simulink model "IC74181Model"  (R2022b)
settings: Solver=VariableStepAuto  StartTime=0.0  StopTime=10.0  RelTol=1e-3
settings Model: Creator=OmerFarukCanbaz  LastModifiedBy=OmerFarukCanbaz

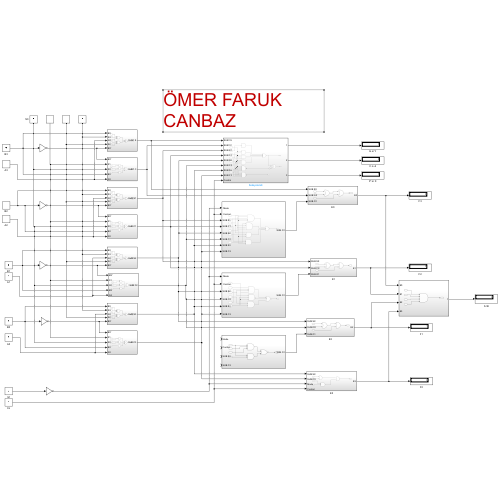
[thumbnail: Simulink's stored preview of the top-level diagram]
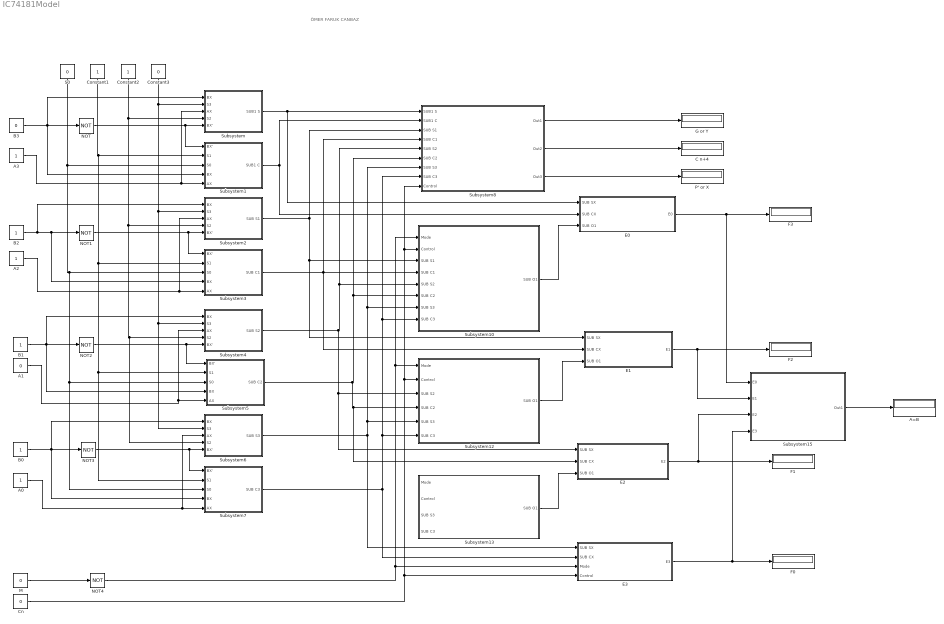
== system IC74181Model ==
  note: ÖMER FARUK CANBAZ
  A0 : Constant
  A1 : Constant  Value=0
  A2 : Constant
  A3 : Constant
  A=B : Display
  B0 : Constant
  B1 : Constant
  B2 : Constant
  B3 : Constant  Value=0
  C n+4 : Display
  Cn : Constant  Value=0
  Constant1 : Constant
  Constant2 : Constant
  Constant3 : Constant  Value=0
  E0 : Subsystem
  E1 : Subsystem
  E2 : Subsystem
  E3 : Subsystem
  F{0..3} (4 alike) : Display
  G or Y : Display
  M : Constant  Value=0
  NOT{,1..4} (5 alike) : Logic  Operator=NOT  IconShape=distinctive  AllPortsSameDT=off  OutDataTypeStr=boolean
  P' or X : Display
  S0 : Constant  Value=0
  Subsystem : Subsystem
  Subsystem1 : Subsystem
  Subsystem10 : Subsystem
  Subsystem12 : Subsystem
  Subsystem13 : Subsystem
  Subsystem15 : Subsystem
  Subsystem2 : Subsystem
  Subsystem3 : Subsystem
  Subsystem4 : Subsystem
  Subsystem5 : Subsystem
  Subsystem6 : Subsystem
  Subsystem7 : Subsystem
  Subsystem8 : Subsystem
  wires:
  B3/1 -> Subsystem/1(BX), NOT/1, Subsystem1/4(BX)
  NOT/1 -> Subsystem1/1(BX'), Subsystem/5(BX')
  A3/1 -> Subsystem/3(AX), Subsystem1/5(AX)
  NOT1/1 -> Subsystem3/1(BX'), Subsystem2/5(BX')
  NOT2/1 -> Subsystem5/1(BX'), Subsystem4/5(BX')
  NOT3/1 -> Subsystem7/1(BX'), Subsystem6/5(BX')
  B2/1 -> Subsystem3/4(BX), NOT1/1, Subsystem2/1(BX)
  A2/1 -> Subsystem2/3(AX), Subsystem3/5(AX)
  B1/1 -> NOT2/1, Subsystem5/4(BX), Subsystem4/1(BX)
  A1/1 -> Subsystem4/3(AX), Subsystem5/5(AX)
  B0/1 -> Subsystem7/4(BX), Subsystem6/1(BX), NOT3/1
  A0/1 -> Subsystem6/3(AX), Subsystem7/5(AX)
  Constant3/1 -> Subsystem6/2(S3), Subsystem4/2(S3), Subsystem2/2(S3), Subsystem/2(S3)
  Constant2/1 -> Subsystem6/4(S2), Subsystem4/4(S2), Subsystem2/4(S2), Subsystem/4(S2)
  Constant1/1 -> Subsystem7/2(S1), Subsystem5/2(S1), Subsystem3/2(S1), Subsystem1/2(S1)
  S0/1 -> Subsystem7/3(S0), Subsystem5/3(S0), Subsystem3/3(S0), Subsystem1/3(S0)
  Subsystem8/1(Out1) -> G or Y/1
  Subsystem8/2(Out2) -> C n+4/1
  Subsystem8/3(Out3) -> P' or X/1
  Subsystem/1(SUB1 S) -> E0/1(SUB SX), Subsystem8/1(SUB1 S)
  Subsystem1/1(SUB1 C) -> Subsystem8/2(SUB1 C), E0/2(SUB CX)
  Subsystem2/1(SUB S1) -> E1/1(SUB SX), Subsystem10/3(SUB S1), Subsystem8/3(SUB S1)
  Subsystem3/1(SUB C1) -> E1/2(SUB CX), Subsystem8/4(SUB C1), Subsystem10/4(SUB C1)
  Subsystem4/1(SUB S2) -> E2/1(SUB SX), Subsystem12/3(SUB S2), Subsystem8/5(SUB S2), Subsystem10/5(SUB S2)
  Subsystem5/1(SUB C2) -> E2/2(SUB CX), Subsystem12/4(SUB C2), Subsystem8/6(SUB C2), Subsystem10/6(SUB C2)
  Subsystem6/1(SUB S3) -> E3/1(SUB SX), Subsystem8/7(SUB S3), Subsystem10/7(SUB S3), Subsystem12/5(SUB S3)
  Subsystem7/1(SUB C3) -> Subsystem12/6(SUB C3), Subsystem8/8(SUB C3), Subsystem10/8(SUB C3), E3/2(SUB CX)
  Cn/1 -> E3/4(Control), Subsystem8/9(Control), Subsystem10/2(" Control"), Subsystem12/2(" Control")
  Subsystem10/1(SUB O1) -> E0/3(SUB O1)
  M/1 -> NOT4/1
  E0/1(E0) -> F3/1, Subsystem15/1(E0)
  NOT4/1 -> E3/3(Mode), Subsystem12/1(" Mode"), Subsystem10/1(" Mode")
  Subsystem12/1(SUB O1) -> E1/3(SUB O1)
  E1/1(E1) -> Subsystem15/2(E1), F2/1
  Subsystem13/1(SUB O1) -> E2/3(SUB O1)
  E2/1(E2) -> F1/1, Subsystem15/3(E2)
  E3/1(E3) -> Subsystem15/4(E3), F0/1
  Subsystem15/1(Out1) -> A=B/1

== system IC74181Model/E0 ==
  SUB SX : Inport
  SUB CX : Inport  Port=2
  SUB O1 : Inport  Port=3
  XOR : Logic  Operator=XOR  IconShape=distinctive  AllPortsSameDT=off  OutDataTypeStr=boolean
  XOR1 : Logic  Operator=XOR  IconShape=distinctive  AllPortsSameDT=off  OutDataTypeStr=boolean
  E0 : Outport
  wires:
  SUB CX/1 -> XOR/2
  SUB SX/1 -> XOR/1
  XOR/1 -> XOR1/1
  SUB O1/1 -> XOR1/2
  XOR1/1 -> E0/1

== system IC74181Model/E1 ==
  SUB SX : Inport
  SUB CX : Inport  Port=2
  SUB O1 : Inport  Port=3
  XOR : Logic  Operator=XOR  IconShape=distinctive  AllPortsSameDT=off  OutDataTypeStr=boolean
  XOR1 : Logic  Operator=XOR  IconShape=distinctive  AllPortsSameDT=off  OutDataTypeStr=boolean
  E1 : Outport
  wires:
  SUB CX/1 -> XOR/2
  SUB SX/1 -> XOR/1
  XOR/1 -> XOR1/1
  SUB O1/1 -> XOR1/2
  XOR1/1 -> E1/1

== system IC74181Model/E2 ==
  SUB SX : Inport
  SUB CX : Inport  Port=2
  SUB O1 : Inport  Port=3
  XOR : Logic  Operator=XOR  IconShape=distinctive  AllPortsSameDT=off  OutDataTypeStr=boolean
  XOR1 : Logic  Operator=XOR  IconShape=distinctive  AllPortsSameDT=off  OutDataTypeStr=boolean
  E2 : Outport
  wires:
  SUB CX/1 -> XOR/2
  SUB SX/1 -> XOR/1
  XOR/1 -> XOR1/1
  SUB O1/1 -> XOR1/2
  XOR1/1 -> E2/1

== system IC74181Model/E3 ==
  SUB SX : Inport
  SUB CX : Inport  Port=2
  Mode : Inport  Port=3
  Control : Inport  Port=4
  NAND : Logic  Operator=NAND  IconShape=distinctive  AllPortsSameDT=off  OutDataTypeStr=boolean
  XOR : Logic  Operator=XOR  IconShape=distinctive  AllPortsSameDT=off  OutDataTypeStr=boolean
  XOR1 : Logic  Operator=XOR  IconShape=distinctive  AllPortsSameDT=off  OutDataTypeStr=boolean
  E3 : Outport
  wires:
  SUB CX/1 -> XOR/2
  SUB SX/1 -> XOR/1
  XOR/1 -> XOR1/1
  Mode/1 -> NAND/1
  XOR1/1 -> E3/1
  Control/1 -> NAND/2
  NAND/1 -> XOR1/2

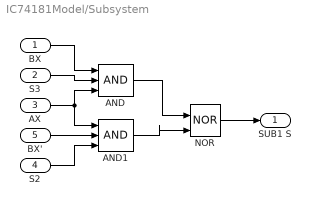
== system IC74181Model/Subsystem ==
  BX : Inport
  S3 : Inport  Port=2
  AX : Inport  Port=3
  S2 : Inport  Port=4
  BX' : Inport  Port=5
  AND : Logic  Inputs=3  IconShape=distinctive  AllPortsSameDT=off  OutDataTypeStr=boolean
  AND1 : Logic  Inputs=3  IconShape=distinctive  AllPortsSameDT=off  OutDataTypeStr=boolean
  NOR : Logic  Operator=NOR  IconShape=distinctive  AllPortsSameDT=off  OutDataTypeStr=boolean
  SUB1 S : Outport
  wires:
  NOR/1 -> SUB1 S/1
  AND1/1 -> NOR/2
  AND/1 -> NOR/1
  AX/1 -> AND1/1, AND/3
  S3/1 -> AND/2
  BX/1 -> AND/1
  S2/1 -> AND1/3
  BX'/1 -> AND1/2

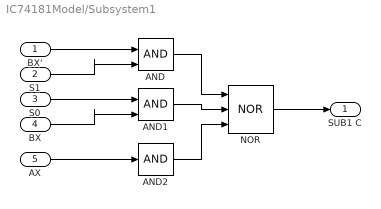
== system IC74181Model/Subsystem1 ==
  BX' : Inport
  S1 : Inport  Port=2
  S0 : Inport  Port=3
  BX : Inport  Port=4
  AX : Inport  Port=5
  AND : Logic  IconShape=distinctive  AllPortsSameDT=off  OutDataTypeStr=boolean
  AND1 : Logic  IconShape=distinctive  AllPortsSameDT=off  OutDataTypeStr=boolean
  AND2 : Logic  Inputs=1  IconShape=distinctive  AllPortsSameDT=off  OutDataTypeStr=boolean
  NOR : Logic  Operator=NOR  Inputs=3  IconShape=distinctive  AllPortsSameDT=off  OutDataTypeStr=boolean
  SUB1 C : Outport
  wires:
  NOR/1 -> SUB1 C/1
  AND/1 -> NOR/1
  AND1/1 -> NOR/2
  AND2/1 -> NOR/3
  AX/1 -> AND2/1
  S0/1 -> AND1/1
  BX/1 -> AND1/2
  S1/1 -> AND/2
  BX'/1 -> AND/1

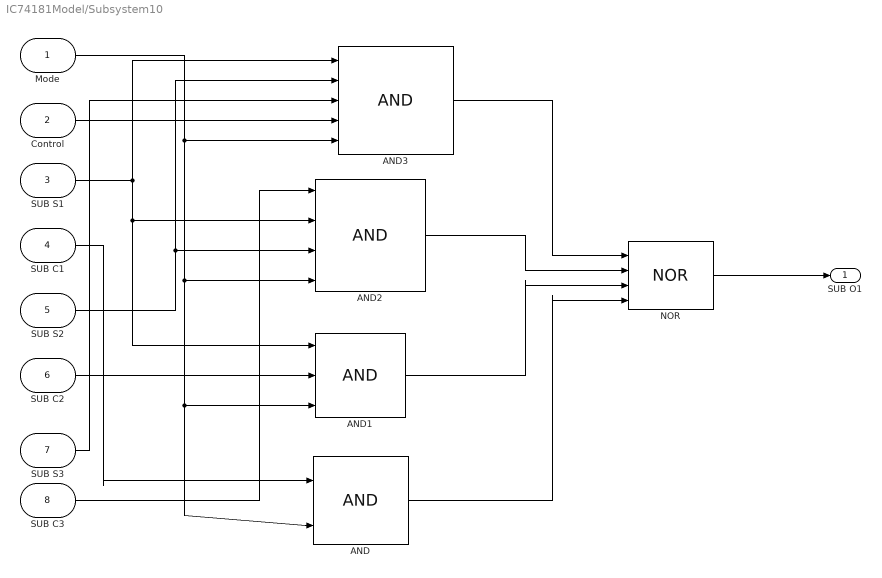
== system IC74181Model/Subsystem10 ==
  " Mode" : Inport
  " Control" : Inport  Port=2
  SUB S1 : Inport  Port=3
  SUB C1 : Inport  Port=4
  SUB S2 : Inport  Port=5
  SUB C2 : Inport  Port=6
  SUB S3 : Inport  Port=7
  SUB C3 : Inport  Port=8
  AND : Logic  IconShape=distinctive  AllPortsSameDT=off  OutDataTypeStr=boolean
  AND1 : Logic  Inputs=3  IconShape=distinctive  AllPortsSameDT=off  OutDataTypeStr=boolean
  AND2 : Logic  Inputs=4  IconShape=distinctive  AllPortsSameDT=off  OutDataTypeStr=boolean
  AND3 : Logic  Inputs=5  IconShape=distinctive  AllPortsSameDT=off  OutDataTypeStr=boolean
  NOR : Logic  Operator=NOR  Inputs=4  IconShape=distinctive  AllPortsSameDT=off  OutDataTypeStr=boolean
  SUB O1 : Outport
  wires:
  AND3/1 -> NOR/1
  AND2/1 -> NOR/2
  AND1/1 -> NOR/3
  AND/1 -> NOR/4
  SUB C1/1 -> AND/1
  " Mode"/1 -> AND2/4, AND/2, AND1/3, AND3/5
  " Control"/1 -> AND3/4
  SUB S3/1 -> AND3/3
  SUB S2/1 -> AND3/2, AND2/3
  SUB C2/1 -> AND1/2
  SUB S1/1 -> AND1/1, AND2/2, AND3/1
  SUB C3/1 -> AND2/1
  NOR/1 -> SUB O1/1

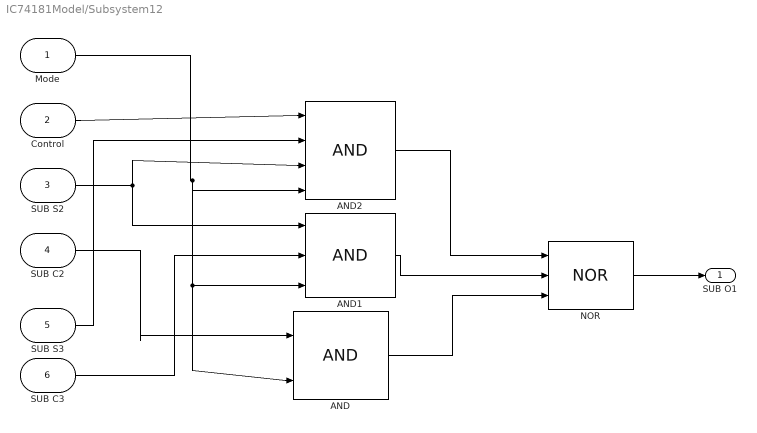
== system IC74181Model/Subsystem12 ==
  " Mode" : Inport
  " Control" : Inport  Port=2
  SUB S2 : Inport  Port=3
  SUB C2 : Inport  Port=4
  SUB S3 : Inport  Port=5
  SUB C3 : Inport  Port=6
  AND : Logic  IconShape=distinctive  AllPortsSameDT=off  OutDataTypeStr=boolean
  AND1 : Logic  Inputs=3  IconShape=distinctive  AllPortsSameDT=off  OutDataTypeStr=boolean
  AND2 : Logic  Inputs=4  IconShape=distinctive  AllPortsSameDT=off  OutDataTypeStr=boolean
  NOR : Logic  Operator=NOR  Inputs=3  IconShape=distinctive  AllPortsSameDT=off  OutDataTypeStr=boolean
  SUB O1 : Outport
  wires:
  NOR/1 -> SUB O1/1
  AND/1 -> NOR/3
  AND1/1 -> NOR/2
  AND2/1 -> NOR/1
  " Mode"/1 -> AND/2, AND1/3, AND2/4
  " Control"/1 -> AND2/1
  SUB S2/1 -> AND1/1, AND2/3
  SUB C2/1 -> AND/1
  SUB C3/1 -> AND1/2
  SUB S3/1 -> AND2/2

== system IC74181Model/Subsystem13 ==
  Mode : Inport
  Control : Inport  Port=2
  SUB S3 : Inport  Port=3
  SUB C3 : Inport  Port=4
  AND : Logic  Inputs=3  IconShape=distinctive  AllPortsSameDT=off  OutDataTypeStr=boolean
  AND1 : Logic  IconShape=distinctive  AllPortsSameDT=off  OutDataTypeStr=boolean
  NOR : Logic  Operator=NOR  IconShape=distinctive  AllPortsSameDT=off  OutDataTypeStr=boolean
  SUB O1 : Outport
  wires:
  Mode/1 -> AND1/1, AND/1
  Control/1 -> AND/2
  SUB S3/1 -> AND/3
  SUB C3/1 -> AND1/2
  NOR/1 -> SUB O1/1
  AND1/1 -> NOR/2
  AND/1 -> NOR/1

== system IC74181Model/Subsystem15 ==
  E0 : Inport
  E1 : Inport  Port=2
  E2 : Inport  Port=3
  E3 : Inport  Port=4
  AND : Logic  Inputs=4  IconShape=distinctive  AllPortsSameDT=off  OutDataTypeStr=boolean
  Out1 : Outport
  wires:
  E3/1 -> AND/4
  E2/1 -> AND/3
  E1/1 -> AND/2
  E0/1 -> AND/1
  AND/1 -> Out1/1

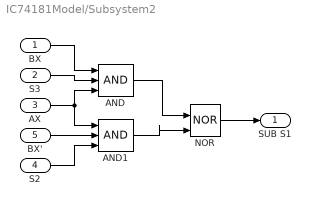
== system IC74181Model/Subsystem2 ==
  BX : Inport
  S3 : Inport  Port=2
  AX : Inport  Port=3
  S2 : Inport  Port=4
  BX' : Inport  Port=5
  AND : Logic  Inputs=3  IconShape=distinctive  AllPortsSameDT=off  OutDataTypeStr=boolean
  AND1 : Logic  Inputs=3  IconShape=distinctive  AllPortsSameDT=off  OutDataTypeStr=boolean
  NOR : Logic  Operator=NOR  IconShape=distinctive  AllPortsSameDT=off  OutDataTypeStr=boolean
  SUB S1 : Outport
  wires:
  NOR/1 -> SUB S1/1
  AND1/1 -> NOR/2
  AND/1 -> NOR/1
  AX/1 -> AND1/1, AND/3
  S3/1 -> AND/2
  BX/1 -> AND/1
  S2/1 -> AND1/3
  BX'/1 -> AND1/2

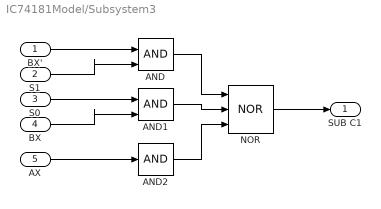
== system IC74181Model/Subsystem3 ==
  BX' : Inport
  S1 : Inport  Port=2
  S0 : Inport  Port=3
  BX : Inport  Port=4
  AX : Inport  Port=5
  AND : Logic  IconShape=distinctive  AllPortsSameDT=off  OutDataTypeStr=boolean
  AND1 : Logic  IconShape=distinctive  AllPortsSameDT=off  OutDataTypeStr=boolean
  AND2 : Logic  Inputs=1  IconShape=distinctive  AllPortsSameDT=off  OutDataTypeStr=boolean
  NOR : Logic  Operator=NOR  Inputs=3  IconShape=distinctive  AllPortsSameDT=off  OutDataTypeStr=boolean
  SUB C1 : Outport
  wires:
  NOR/1 -> SUB C1/1
  AND/1 -> NOR/1
  AND1/1 -> NOR/2
  AND2/1 -> NOR/3
  AX/1 -> AND2/1
  S0/1 -> AND1/1
  BX/1 -> AND1/2
  S1/1 -> AND/2
  BX'/1 -> AND/1

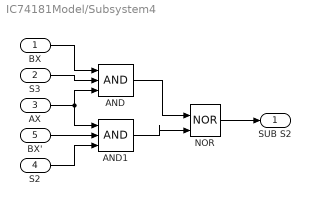
== system IC74181Model/Subsystem4 ==
  BX : Inport
  S3 : Inport  Port=2
  AX : Inport  Port=3
  S2 : Inport  Port=4
  BX' : Inport  Port=5
  AND : Logic  Inputs=3  IconShape=distinctive  AllPortsSameDT=off  OutDataTypeStr=boolean
  AND1 : Logic  Inputs=3  IconShape=distinctive  AllPortsSameDT=off  OutDataTypeStr=boolean
  NOR : Logic  Operator=NOR  IconShape=distinctive  AllPortsSameDT=off  OutDataTypeStr=boolean
  SUB S2 : Outport
  wires:
  NOR/1 -> SUB S2/1
  AND1/1 -> NOR/2
  AND/1 -> NOR/1
  AX/1 -> AND1/1, AND/3
  S3/1 -> AND/2
  BX/1 -> AND/1
  S2/1 -> AND1/3
  BX'/1 -> AND1/2

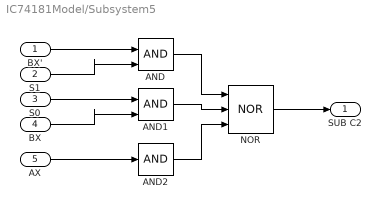
== system IC74181Model/Subsystem5 ==
  BX' : Inport
  S1 : Inport  Port=2
  S0 : Inport  Port=3
  BX : Inport  Port=4
  AX : Inport  Port=5
  AND : Logic  IconShape=distinctive  AllPortsSameDT=off  OutDataTypeStr=boolean
  AND1 : Logic  IconShape=distinctive  AllPortsSameDT=off  OutDataTypeStr=boolean
  AND2 : Logic  Inputs=1  IconShape=distinctive  AllPortsSameDT=off  OutDataTypeStr=boolean
  NOR : Logic  Operator=NOR  Inputs=3  IconShape=distinctive  AllPortsSameDT=off  OutDataTypeStr=boolean
  SUB C2 : Outport
  wires:
  NOR/1 -> SUB C2/1
  AND/1 -> NOR/1
  AND1/1 -> NOR/2
  AND2/1 -> NOR/3
  AX/1 -> AND2/1
  S0/1 -> AND1/1
  BX/1 -> AND1/2
  S1/1 -> AND/2
  BX'/1 -> AND/1

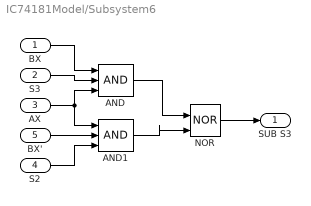
== system IC74181Model/Subsystem6 ==
  BX : Inport
  S3 : Inport  Port=2
  AX : Inport  Port=3
  S2 : Inport  Port=4
  BX' : Inport  Port=5
  AND : Logic  Inputs=3  IconShape=distinctive  AllPortsSameDT=off  OutDataTypeStr=boolean
  AND1 : Logic  Inputs=3  IconShape=distinctive  AllPortsSameDT=off  OutDataTypeStr=boolean
  NOR : Logic  Operator=NOR  IconShape=distinctive  AllPortsSameDT=off  OutDataTypeStr=boolean
  SUB S3 : Outport
  wires:
  NOR/1 -> SUB S3/1
  AND1/1 -> NOR/2
  AND/1 -> NOR/1
  AX/1 -> AND1/1, AND/3
  S3/1 -> AND/2
  BX/1 -> AND/1
  S2/1 -> AND1/3
  BX'/1 -> AND1/2

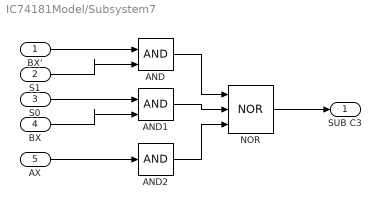
== system IC74181Model/Subsystem7 ==
  BX' : Inport
  S1 : Inport  Port=2
  S0 : Inport  Port=3
  BX : Inport  Port=4
  AX : Inport  Port=5
  AND : Logic  IconShape=distinctive  AllPortsSameDT=off  OutDataTypeStr=boolean
  AND1 : Logic  IconShape=distinctive  AllPortsSameDT=off  OutDataTypeStr=boolean
  AND2 : Logic  Inputs=1  IconShape=distinctive  AllPortsSameDT=off  OutDataTypeStr=boolean
  NOR : Logic  Operator=NOR  Inputs=3  IconShape=distinctive  AllPortsSameDT=off  OutDataTypeStr=boolean
  SUB C3 : Outport
  wires:
  NOR/1 -> SUB C3/1
  AND/1 -> NOR/1
  AND1/1 -> NOR/2
  AND2/1 -> NOR/3
  AX/1 -> AND2/1
  S0/1 -> AND1/1
  BX/1 -> AND1/2
  S1/1 -> AND/2
  BX'/1 -> AND/1

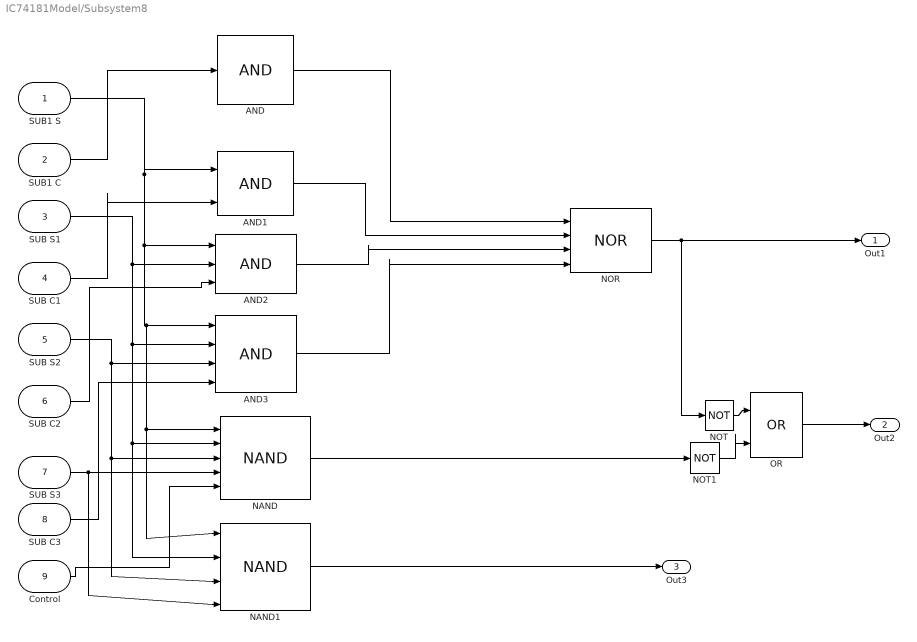
== system IC74181Model/Subsystem8 ==
  SUB1 S : Inport
  SUB1 C : Inport  Port=2
  SUB S1 : Inport  Port=3
  SUB C1 : Inport  Port=4
  SUB S2 : Inport  Port=5
  SUB C2 : Inport  Port=6
  SUB S3 : Inport  Port=7
  SUB C3 : Inport  Port=8
  Control : Inport  Port=9
  AND : Logic  Inputs=1  IconShape=distinctive  AllPortsSameDT=off  OutDataTypeStr=boolean
  AND1 : Logic  IconShape=distinctive  AllPortsSameDT=off  OutDataTypeStr=boolean
  AND2 : Logic  Inputs=3  IconShape=distinctive  AllPortsSameDT=off  OutDataTypeStr=boolean
  AND3 : Logic  Inputs=4  IconShape=distinctive  AllPortsSameDT=off  OutDataTypeStr=boolean
  NAND : Logic  Operator=NAND  Inputs=5  IconShape=distinctive  AllPortsSameDT=off  OutDataTypeStr=boolean
  NAND1 : Logic  Operator=NAND  Inputs=4  IconShape=distinctive  AllPortsSameDT=off  OutDataTypeStr=boolean
  NOR : Logic  Operator=NOR  Inputs=4  IconShape=distinctive  AllPortsSameDT=off  OutDataTypeStr=boolean
  NOT : Logic  Operator=NOT  IconShape=distinctive  AllPortsSameDT=off  OutDataTypeStr=boolean
  NOT1 : Logic  Operator=NOT  IconShape=distinctive  AllPortsSameDT=off  OutDataTypeStr=boolean
  OR : Logic  Operator=OR  IconShape=distinctive  AllPortsSameDT=off  OutDataTypeStr=boolean
  Out1 : Outport
  Out2 : Outport  Port=2
  Out3 : Outport  Port=3
  wires:
  NAND1/1 -> Out3/1
  OR/1 -> Out2/1
  NOT/1 -> OR/1
  NOT1/1 -> OR/2
  NAND/1 -> NOT1/1
  NOR/1 -> NOT/1, Out1/1
  SUB1 S/1 -> NAND1/1, NAND/1, AND3/1, AND2/1, AND1/1
  AND/1 -> NOR/1
  AND1/1 -> NOR/2
  AND2/1 -> NOR/3
  AND3/1 -> NOR/4
  SUB1 C/1 -> AND/1
  SUB C1/1 -> AND1/2
  SUB S1/1 -> NAND1/2, NAND/2, AND3/2, AND2/2
  SUB C2/1 -> AND2/3
  SUB S2/1 -> NAND1/3, NAND/3, AND3/3
  SUB C3/1 -> AND3/4
  SUB S3/1 -> NAND1/4, NAND/4
  Control/1 -> NAND/5
